simulink model "asadi_simulation"  (R2024b)
settings: Solver=VariableStepAuto  StartTime=0.0  StopTime=10  FixedStep=0.01  RelTol=1e-3
model workspace (MAT data in the model file):
  I_L = Simulink.Parameter
  I_L.Value = 0.0696
  I_L.Complexity = 'real'
  I_L.Dimensions = [1 1]
  I_L.DataType = 'auto'
  L = Simulink.Parameter
  L.Value = 0.375
  L.Complexity = 'real'
  L.Dimensions = [1 1]
  L.DataType = 'auto'
  M_EE = Simulink.Parameter
  M_EE.Value = 1.542
  M_EE.Complexity = 'real'
  M_EE.Dimensions = [1 1]
  M_EE.DataType = 'auto'
  M_L = Simulink.Parameter
  M_L.Value = 1.696
  M_L.Complexity = 'real'
  M_L.Dimensions = [1 1]
  M_L.DataType = 'auto'
  M_l = Simulink.Parameter
  M_l.Value = 0.334
  M_l.Complexity = 'real'
  M_l.Dimensions = [1 1]
  M_l.DataType = 'auto'
  l = Simulink.Parameter
  l.Value = 0.96
  l.Complexity = 'real'
  l.Dimensions = [1 1]
  l.DataType = 'auto'
undefined symbols (not defined in the file): i_L, l_L, l_l, m_EE, m_L, m_l
libraries: simulink x3
settings Model: Creator=marius  LastModifiedBy=marius
settings RTWCC: GPUComputeCapability=3.5

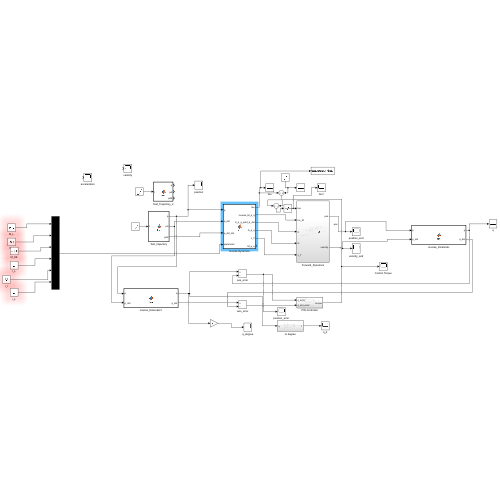
[thumbnail: Simulink's stored preview of the top-level diagram]
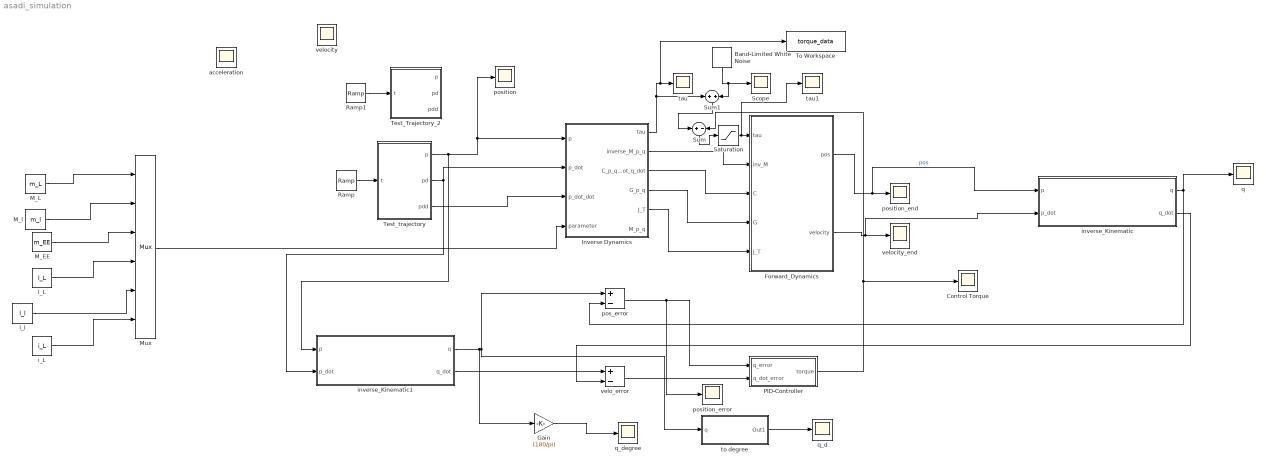
== system asadi_simulation ==
  Band-Limited White Noise : simulink/Sources/Band-Limited White Noise  Cov=[0.0005]  Ts=0.1  seed=[23341]
  Control Torque : Scope
  Forward_Dynamics : Subsystem
  Gain : Gain  Gain=(180/pi)
  Inverse Dynamics : MATLAB Function  TreatAsAtomicUnit=on
  M_EE : Constant  Value=m_EE
  M_L : Constant  Value=m_L
  M_l : Constant  Value=m_l
  Mux : Mux  Inputs=6
  PID-Controller : Subsystem
  Ramp : simulink/Sources/Ramp  slope=1  start=0  InitialOutput=0
  Ramp1 : simulink/Sources/Ramp  slope=1  start=0  InitialOutput=0
  Saturation : Saturate  UpperLimit=26  LowerLimit=-26
  Scope : Scope
  Sum : Sum  Inputs=+-
  Sum1 : Sum
  Test_Trajectory_2 : MATLAB Function  TreatAsAtomicUnit=on
  Test_trajectory : MATLAB Function  TreatAsAtomicUnit=on
  To Workspace : ToWorkspace  VariableName=torque_data  SaveFormat=Timeseries  SampleTime=-1
  acceleration : Scope
  i_L : Constant  Value=i_L
  inverse_Kinematic : MATLAB Function  TreatAsAtomicUnit=on
  inverse_Kinematic1 : MATLAB Function  TreatAsAtomicUnit=on
  l_L : Constant  Value=l_L
  l_l : Constant  Value=l_l
  pos_error : Sum  Inputs=+-
  position : Scope
  position_end : Scope
  position_error : Scope
  q : Scope
  q_d : Scope
  q_degree : Scope
  tau : Scope
  tau1 : Scope
  to degree : Subsystem
  velo_error : Sum  Inputs=+-
  velocity : Scope
  velocity_end : Scope
  wires:
  Inverse Dynamics/1(tau) -> Sum1/1, To Workspace/1, tau/1
  Inverse Dynamics/2(inverse_M_p_q) -> Forward_Dynamics/2(inv_M)
  Inverse Dynamics/3(C_p_q_pdot_q_dot) -> Forward_Dynamics/3(C)
  Inverse Dynamics/4(G_p_q) -> Forward_Dynamics/4(G)
  Inverse Dynamics/5(J_T) -> Forward_Dynamics/5(J_T)
  Forward_Dynamics/1(pos) -> inverse_Kinematic/1(p), position_end/1  "pos"
  Forward_Dynamics/2(velocity) -> inverse_Kinematic/2(p_dot), velocity_end/1
  pos_error/1 -> position_error/1, PID-Controller/1(q_error)
  inverse_Kinematic1/2(q_dot) -> velo_error/1
  inverse_Kinematic/2(q_dot) -> velo_error/2
  inverse_Kinematic/1(q) -> q/1, pos_error/2
  inverse_Kinematic1/1(q) -> Gain/1, pos_error/1, to degree/1(q)
  velo_error/1 -> PID-Controller/2(q_dot_error)
  Gain/1 -> q_degree/1
  Band-Limited White Noise/1 -> Scope/1, Sum1/2
  Sum1/1 -> Sum/1
  Ramp/1 -> Test_trajectory/1(t)
  Sum/1 -> Saturation/1
  to degree/1(Out1) -> q_d/1
  Saturation/1 -> tau1/1, Forward_Dynamics/1(tau)
  PID-Controller/1(torque) -> Sum/2, Control Torque/1
  Ramp1/1 -> Test_Trajectory_2/1(t)
  Test_trajectory/1(p) -> inverse_Kinematic1/1(p), position/1, Inverse Dynamics/1(p)
  Test_trajectory/2(pd) -> inverse_Kinematic1/2(p_dot), Inverse Dynamics/2(p_dot)
  Test_trajectory/3(pdd) -> Inverse Dynamics/3(p_dot_dot)
  M_L/1 -> Mux/1
  M_l/1 -> Mux/2
  M_EE/1 -> Mux/3
  Mux/1 -> Inverse Dynamics/4(parameter)
  l_L/1 -> Mux/4
  l_l/1 -> Mux/5
  i_L/1 -> Mux/6

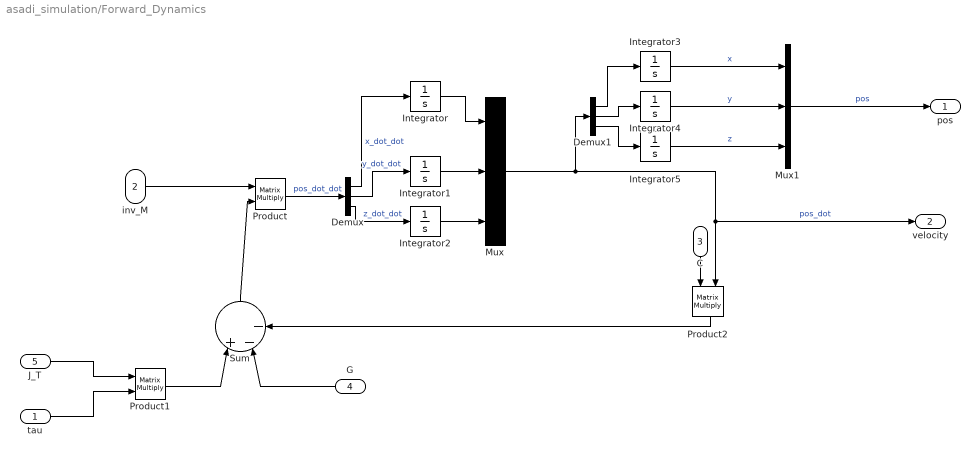
== system asadi_simulation/Forward_Dynamics ==
  tau : Inport
  inv_M : Inport  Port=2
  C : Inport  Port=3
  G : Inport  Port=4
  J_T : Inport  Port=5
  Demux : Demux  Outputs=3
  Demux1 : Demux  Outputs=3
  Integrator : Integrator  InitialCondition=0.4
  Integrator1 : Integrator  InitialCondition=0.8
  Integrator2 : Integrator  InitialCondition=0.8
  Integrator3 : Integrator
  Integrator4 : Integrator
  Integrator5 : Integrator  InitialCondition=-0.9
  Mux : Mux  Inputs=3
  Mux1 : Mux  Inputs=3
  Product : Product  Multiplication=Matrix(*)
  Product1 : Product  Multiplication=Matrix(*)
  Product2 : Product  Multiplication=Matrix(*)
  Sum : Sum  Inputs=|+--
  pos : Outport
  velocity : Outport  Port=2
  wires:
  inv_M/1 -> Product/1
  J_T/1 -> Product1/1
  tau/1 -> Product1/2
  Product1/1 -> Sum/1
  G/1 -> Sum/2
  Product2/1 -> Sum/3
  Sum/1 -> Product/2
  Product/1 -> Demux/1  "pos_dot_dot"
  Demux/3 -> Integrator2/1  "z_dot_dot"
  Demux/2 -> Integrator1/1  "y_dot_dot"
  Demux/1 -> Integrator/1  "x_dot_dot"
  Integrator2/1 -> Mux/3
  Integrator1/1 -> Mux/2
  Integrator/1 -> Mux/1
  Mux/1 -> velocity/1, Product2/2, Demux1/1  "pos_dot"
  Demux1/3 -> Integrator5/1
  Demux1/2 -> Integrator4/1
  Demux1/1 -> Integrator3/1
  Integrator5/1 -> Mux1/3  "z"
  Integrator4/1 -> Mux1/2  "y"
  Integrator3/1 -> Mux1/1  "x"
  Mux1/1 -> pos/1  "pos"
  C/1 -> Product2/1

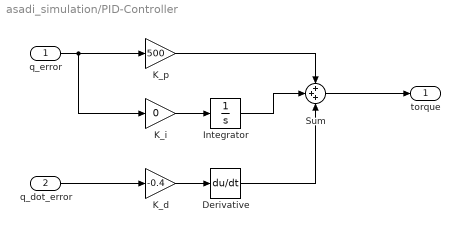
== system asadi_simulation/PID-Controller ==
  q_error : Inport
  q_dot_error : Inport  Port=2
  Derivative : Derivative
  Integrator : Integrator
  K_d : Gain  Gain=-0.4
  K_i : Gain  Gain=0
  K_p : Gain  Gain=500
  Sum : Sum  Inputs=+++
  torque : Outport
  wires:
  q_error/1 -> K_i/1, K_p/1
  K_p/1 -> Sum/1
  K_i/1 -> Integrator/1
  Integrator/1 -> Sum/2
  q_dot_error/1 -> K_d/1
  K_d/1 -> Derivative/1
  Derivative/1 -> Sum/3
  Sum/1 -> torque/1

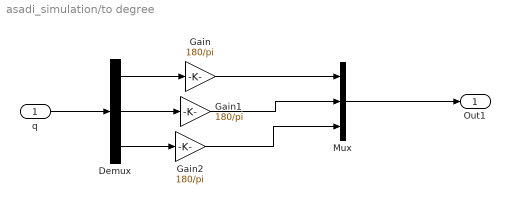
== system asadi_simulation/to degree ==
  q : Inport
  Demux : Demux  Outputs=3
  Gain : Gain  Gain=180/pi
  Gain1 : Gain  Gain=180/pi
  Gain2 : Gain  Gain=180/pi
  Mux : Mux  Inputs=3
  Out1 : Outport
  wires:
  q/1 -> Demux/1
  Demux/3 -> Gain2/1
  Gain2/1 -> Mux/3
  Demux/2 -> Gain1/1
  Demux/1 -> Gain/1
  Gain/1 -> Mux/1
  Gain1/1 -> Mux/2
  Mux/1 -> Out1/1

== matlab function asadi_simulation/Test_trajectory ==
  data: t input; p output; pd output; pdd output
function [p, pd, pdd] = fcn(t)
pos_x= sin(2*t) * 0.2;
pos_y= sin(4*t) * 0.2;
pos_z = -0.9 + sin (4*t) * 0.2;
vel_x = 0.4 * cos(2*t);
vel_y = 0.8 * cos(4*t);
vel_z = cos(4*t) * 0.8;
acc_x = -0.8 * sin(2*t);
acc_y = -3.2*sin(4*t);
acc_z = -3.2 * sin(4*t);

p= [pos_x; pos_y; pos_z];
pd = [vel_x; vel_y; vel_z];
pdd = [acc_x; acc_y; acc_z];

== matlab function asadi_simulation/Inverse Dynamics ==
  data: p input; tau output; p_dot input; p_dot_dot input; inverse_M_p_q output; C_p_q_pdot_q_dot output; G_p_q output; J_T output; M_p_q output; parameter input
function [tau, inverse_M_p_q, C_p_q_pdot_q_dot, G_p_q, J_T, M_p_q]    = fcn(p, p_dot, p_dot_dot, parameter)
r_p = 0.07; %m
% radius base platform
r_b = 0.25; %m
%length upper arm
L = parameter(4);%0.375; m
%length fore arm
l = parameter(5); %0.96; %m

% mass proximal link
m_L = parameter(1);%1.636 kg
% mass distal link
M_K = parameter(2); %0.334 kg

% mass end_effector
m_p = parameter(3); %1.542kg

%proximal link inertia
I_L = parameter(6);%0.0696 ;% kg m^2

g = [0; 0; -9.808]; % m/s^2
c = r_p - r_b;
x = p(1);
y = p(2);
z = p(3);
E1 = -(x + 2*c + sqrt(3)* y) * L;
E2 = -(x + 2*c - sqrt(3)* y) * L;
E3 = 2*(x-c)*L;

F1 = 2*z*L;
F2 = 2*z*L;
F3 = 2*z*L;

G1 = x^2 + y^2 + z^2 + c*x + c^2 + L^2 + sqrt(3)* c * y - l^2;
G2 = x^2 + y^2 + z^2 + c*x +c^2 + L^2 - sqrt(3)* c * y - l^2;
G3 = x^2 + y^2 + z^2 + c^2 -2*c*x + L^2 -l^2;

auxterm_1 = E1^2 + F1^2 - G1^2;
auxterm_2 = E2^2 + F2^2 - G2^2;
auxterm_3 = E3^2 + F3^2 - G3^2;

t_1_1 = (-F1 + sqrt(auxterm_1)) / (G1 - E1);
t_1_2 = (-F1 - sqrt(auxterm_1)) / (G1 - E1);

t_2_1 = (-F2 + sqrt(auxterm_2)) / (G2 - E2);
t_2_2 = (-F2 - sqrt(auxterm_2)) / (G2 - E2);

t_3_1 = (-F3 + sqrt(auxterm_3)) / (G3 - E3);
t_3_2 = (-F3 - sqrt(auxterm_3)) / (G3 - E3);

theta_1_1 = 2*atan(t_1_1);
theta_1_2 = 2*atan(t_1_2);
theta_1_1_deg = theta_1_1 * 180/pi;
theta_1_2_deg = theta_1_2 * 180/pi;

theta_2_1 = 2*atan(t_2_1);
theta_2_2 = 2*atan(t_2_2);
theta_2_1_deg = theta_2_1 * 180/pi;
theta_2_2_deg = theta_2_2 * 180/pi;

theta_3_1 = 2*atan(t_3_1);
theta_3_2 = 2*atan(t_3_2);
theta_3_1_deg = theta_3_1 * 180/pi;
theta_3_2_deg = theta_3_2 * 180/pi;


q1 = -theta_1_2;
q2 = -theta_2_2;
q3 = -theta_3_2; % minus because asadi uses another convention, q turns in negative direction

% Jacobians

R_b = [0; r_b; 0];
R_a = [0; r_p; 0];

phi_1 = -pi/6;
phi_2 = -5*pi/6;
phi_3 = pi/2;


rotation_R_1 = [cos(phi_1) -sin(phi_1) 0; sin(phi_1) cos(phi_1) 0; 0 0 1];
rotation_R_2 = [cos(phi_2) -sin(phi_2) 0; sin(phi_2) cos(phi_2) 0; 0 0 1];
rotation_R_3 = [cos(phi_3) -sin(phi_3) 0; sin(phi_3) cos(phi_3) 0; 0 0 1];

rotation_O_1 = [1 0 0; 0 cos(q1) -sin(q1); 0 sin(q1) cos(q1)];
rotation_O_2 = [1 0 0; 0 cos(q2) -sin(q2); 0 sin(q2) cos(q2)];
rotation_O_3 = [1 0 0; 0 cos(q3) -sin(q3); 0 sin(q3) cos(q3)];

%L vector along the positive y-Axis of the frame which moves with the upper
%arm
L_vec = [0; L; 0];
U_1 = p - rotation_R_1*((R_b - R_a) + rotation_O_1*L_vec);

U_2 = p - rotation_R_2*((R_b - R_a) + rotation_O_2*L_vec);
U_3 = p - rotation_R_3*((R_b - R_a) + rotation_O_3*L_vec);

S_1 = [0 0 0; 0 0 -1; 0 1 0];
T_1 = rotation_R_1 * S_1 * rotation_O_1* L_vec;
T_2 = rotation_R_2 * S_1 * rotation_O_2* L_vec;
T_3 = rotation_R_3 * S_1 * rotation_O_3* L_vec;


Jacobian = [U_1'*T_1, 0, 0; 0, U_2'*T_2, 0; 0, 0, U_3'*T_3] \ [U_1'; U_2'; U_3'];

%q_dot
q_dot = Jacobian * p_dot;


T_dot_1 = rotation_R_1*S_1 * S_1 * rotation_O_1* L_vec * q_dot(1);
T_dot_2 = rotation_R_2*S_1 * S_1 * rotation_O_2* L_vec * q_dot(2);
T_dot_3 = rotation_R_3*S_1 * S_1 * rotation_O_3* L_vec * q_dot(3);

U_dot_1 = p_dot - T_1 * q_dot(1);
U_dot_2 = p_dot - T_2 * q_dot(2);
U_dot_3 = p_dot - T_3 * q_dot(3);

inverse_Jacobian_aux = inv([U_1'*T_1, 0, 0; 0, U_2'*T_2, 0; 0, 0, U_3'*T_3]);
%another auxiliary vector
vec_1 = U_dot_1' - (U_dot_1' * T_1 + U_1'*T_dot_1)*Jacobian(1,:);
vec_2 = U_dot_2' - (U_dot_2' * T_2 + U_2'*T_dot_2)*Jacobian(2,:);
vec_3 = U_dot_3' - (U_dot_3' * T_3 + U_3'*T_dot_3)*Jacobian(3,:);

Jacobian_dot = cross(inverse_Jacobian_aux, [vec_1; vec_2; vec_3]);

omega_L_1 = [Jacobian(1,:); 0 0 0; 0 0 0] * p_dot;
omega_L_2 = [Jacobian(2,:); 0 0 0; 0 0 0] * p_dot;
omega_L_3 = [Jacobian(3,:); 0 0 0; 0 0 0] * p_dot;

r_L = 0.373; %proximal link length ratio COM
v_L_1 = cross(omega_L_1, r_L*[0;1;0]);
v_L_2 = cross(omega_L_2, r_L*[0;1;0]);
v_L_3 = cross(omega_L_3, r_L*[0;1;0]);

omega_L_dot_1 = [Jacobian(1,:); 0 0 0; 0 0 0]* p_dot_dot + [Jacobian_dot(1,:); 0 0 0; 0 0 0] * p_dot;
omega_L_dot_2 = [Jacobian(2,:); 0 0 0; 0 0 0]* p_dot_dot + [Jacobian_dot(2,:); 0 0 0; 0 0 0] * p_dot;
omega_L_dot_3 = [Jacobian(3,:); 0 0 0; 0 0 0]* p_dot_dot + [Jacobian_dot(3,:); 0 0 0; 0 0 0] * p_dot;

v_L_dot_1 = r_L * L * [0 0 0; 0 0 0; Jacobian(1,:)]* p_dot_dot + r_L * L *...
    [0 0 0; -p_dot' * Jacobian(1, :)' * Jacobian(1,:); Jacobian_dot(1,:)] * p_dot;
v_L_dot_2 = r_L * L * [0 0 0; 0 0 0; Jacobian(2,:)]* p_dot_dot + r_L * L *...
    [0 0 0; -p_dot' * Jacobian(2, :)' * Jacobian(2,:); Jacobian_dot(2,:)] * p_dot;
v_L_dot_3 = r_L * L * [0 0 0; 0 0 0; Jacobian(3,:)]* p_dot_dot + r_L * L *...
    [0 0 0; -p_dot' * Jacobian(3, :)' * Jacobian(3,:); Jacobian_dot(3,:)] * p_dot;
r_K = 0.5; % distal link length ratio COM

v_K_1 = ((1-r_K)*L*[0 0 0; 0 0 0; Jacobian(1,:)] + r_K * rotation_O_1' * rotation_R_1') * p_dot;
v_K_2 = ((1-r_K)*L*[0 0 0; 0 0 0; Jacobian(2,:)] + r_K * rotation_O_2' * rotation_R_2') * p_dot;
v_K_3 = ((1-r_K)*L*[0 0 0; 0 0 0; Jacobian(3,:)] + r_K * rotation_O_3' * rotation_R_3') * p_dot;

v_K_dot_1 = ((1-r_K)*L*[0 0 0; 0 0 0; Jacobian(1,:)] + r_K * rotation_O_1' * rotation_R_1') * p_dot_dot...
    + (1-r_K)* L * [0 0 0; - p_dot' * Jacobian(1,:)' * Jacobian(1,:); Jacobian_dot(1,:)]* p_dot;

v_K_dot_2 = ((1-r_K)*L*[0 0 0; 0 0 0; Jacobian(2,:)] + r_K * rotation_O_2' * rotation_R_2') * p_dot_dot...
    + (1-r_K)* L * [0 0 0; - p_dot' * Jacobian(2,:)' * Jacobian(2,:); Jacobian_dot(2,:)]* p_dot;

v_K_dot_3 = ((1-r_K)*L*[0 0 0; 0 0 0; Jacobian(3,:)] + r_K * rotation_O_3' * rotation_R_3') * p_dot_dot...
    + (1-r_K)* L * [0 0 0; - p_dot' * Jacobian(3,:)' * Jacobian(3,:); Jacobian_dot(3,:)]* p_dot;


% auxiliary Jacobians
J_L_1 = r_L * L * [0 0 0; 0 0 0; Jacobian(1,:)];
J_L_2 = r_L * L * [0 0 0; 0 0 0; Jacobian(2,:)];
J_L_3 = r_L * L * [0 0 0; 0 0 0; Jacobian(3,:)];

J_K_1 = (1-r_K)* L* [0 0 0; 0 0 0; Jacobian(1,:)] + r_K *rotation_O_1' * rotation_R_1';
J_K_2 = (1-r_K)* L* [0 0 0; 0 0 0; Jacobian(2,:)] + r_K *rotation_O_2' * rotation_R_2';
J_K_3 = (1-r_K)* L* [0 0 0; 0 0 0; Jacobian(3,:)] + r_K *rotation_O_3' * rotation_R_3';

J_C_1 = L * [0 0 0; 0 0 0; Jacobian(1,:)];
J_C_2 = L * [0 0 0; 0 0 0; Jacobian(2,:)];
J_C_3 = L * [0 0 0; 0 0 0; Jacobian(3,:)];


% distal link dominant inertia
I_K = 0.00057; %kg m^2
% Inertia motor
I_Mo = 0.0465;


% mass distributions
A = [1 1 1; r_K (r_K-1) 0; r_K^2*l^2 (r_K-1)^2 *l^2 0];
b_vec = [M_K; 0; I_K];
x = A\b_vec;
% mass distributed to elbow
m_c = x(1);
% mass distributed to endeffector
m_A = x(2);
% mass distributed to COM distal link
m_K = x(3);

identity = eye(3);


% Massmatrix 

sum_one = m_K* r_K * J_K_1' * rotation_O_1' * rotation_R_1'...
    + m_K * r_K * J_K_2'*rotation_O_2'* rotation_R_2' + m_K* r_K * J_K_3' * rotation_O_3' * rotation_R_3';
sum_two_one = (m_c*L*J_C_1' + m_L * r_L * L * J_L_1' + m_K*(1-r_K)*L*J_K_1') * [0 0 0; 0 0 0; Jacobian(1,:)];
sum_two_two = (m_c*L*J_C_2' + m_L * r_L * L * J_L_2' + m_K*(1-r_K)*L*J_K_2') * [0 0 0; 0 0 0; Jacobian(2,:)];
sum_two_three = (m_c*L*J_C_3' + m_L * r_L * L * J_L_3' + m_K*(1-r_K)*L*J_K_3') * [0 0 0; 0 0 0; Jacobian(3,:)];
sum_two = sum_two_one + sum_two_two + sum_two_three;
M_p_q = (I_Mo +  I_L) * (Jacobian' * Jacobian) + (m_p + 3*m_c)* identity + sum_one + sum_two;


% matrix of coriolis and centrifugal forces
sum_c = (m_c*L*J_C_1' + m_L*r_L*L * J_L_1' + m_K*(1-r_K)*L*J_K_1') * [0 0 0; -p_dot' *Jacobian(1,:)' * Jacobian(1,:); Jacobian_dot(1,:)]...
    +(m_c*L*J_C_2' + m_L*r_L*L * J_L_2' + m_K*(1-r_K)*L*J_K_2') * [0 0 0; -p_dot' *Jacobian(2,:)' * Jacobian(2,:); Jacobian_dot(2,:)]...
    +(m_c*L*J_C_3' + m_L*r_L*L * J_L_3' + m_K*(1-r_K)*L*J_K_3') * [0 0 0; -p_dot' *Jacobian(3,:)' * Jacobian(3,:); Jacobian_dot(3,:)];
C_p_q_pdot_q_dot = (I_Mo + I_L)* Jacobian' * Jacobian_dot + sum_c;


sum_g = ((m_c* J_C_1' + m_L*J_L_1' + m_K* J_K_1') * rotation_O_1' * rotation_R_1')*g ...
    + ((m_c* J_C_2' + m_L*J_L_2' + m_K* J_K_2') * rotation_O_2' * rotation_R_2')*g ...
    + ((m_c* J_C_3' + m_L*J_L_3' + m_K* J_K_3') * rotation_O_3' * rotation_R_3')*g;

G_p_q = -(m_p + 3* m_A) * g - sum_g;
inverse_M_p_q = inv(M_p_q);
J_T = Jacobian';
F_p = 0;
motion_equation =  M_p_q * p_dot_dot + C_p_q_pdot_q_dot * p_dot + G_p_q - F_p;
tau =  J_T\ motion_equation;

== matlab function asadi_simulation/inverse_Kinematic ==
  data: p input; q output; p_dot input; q_dot output
function [q, q_dot] = fcn(p, p_dot)

% radius moving platform
r_p = 0.07; %m
% radius base platform
r_b = 0.25; %m
%length upper arm
L = 0.375; %m
%length fore arm
l = 0.96; %m

c = r_p - r_b;
x = p(1);
y = p(2);
z = p(3);

E1 = -(x + 2*c + sqrt(3)* y) * L;
E2 = -(x + 2*c - sqrt(3)* y) * L;
E3 = 2*(x-c)*L;

F1 = 2*z*L;
F2 = 2*z*L;
F3 = 2*z*L;

abs_pos = x^2 + y^2 + z^2;
G1 = abs_pos + c*x + c^2 + L^2 + sqrt(3)* c * y - l^2;
G2 = abs_pos + c*x +c^2 + L^2 - sqrt(3)* c * y - l^2;
G3 = abs_pos + c^2 -2*c*x + L^2 -l^2;


%auxiliary term
aux_T_1 = sqrt(E1^2 + F1^2 - G1^2);
aux_T_2 = sqrt(E2^2 + F2^2 - G2^2);
aux_T_3 = sqrt(E3^2 + F3^2 - G3^2);
%quadratic formula.
t_1_1 = (-F1 + aux_T_1) / (G1 - E1);
t_1_2 = (-F1 - aux_T_1) / (G1 - E1);

t_2_1 = (-F2 + aux_T_2) / (G2 - E2);
t_2_2 = (-F2 - aux_T_2) / (G2 - E2);

t_3_1 = (-F3 + aux_T_3) / (G3 - E3);
t_3_2 = (-F3 - aux_T_3) / (G3 - E3);

theta_1_1 = 2*atan(t_1_1);
theta_1_2 = 2*atan(t_1_2);


theta_2_1 = 2*atan(t_2_1);
theta_2_2 = 2*atan(t_2_2);

theta_3_1 = 2*atan(t_3_1);
theta_3_2 = 2*atan(t_3_2);


q1 = -theta_1_2;
q2 = -theta_2_2;
q3 = -theta_3_2;
% using the negative because of different convention
q=-[q1; q2; q3];
% Jacobians

R_b = [0; r_b; 0];
R_a = [0; r_p; 0];
phi_1 = -pi/6;
phi_2 = -5*pi/6;
phi_3 = pi/2;
rotation_R_1 = [cos(phi_1) -sin(phi_1) 0; sin(phi_1) cos(phi_1) 0; 0 0 1];
rotation_R_2 = [cos(phi_2) -sin(phi_2) 0; sin(phi_2) cos(phi_2) 0; 0 0 1];
rotation_R_3 = [cos(phi_3) -sin(phi_3) 0; sin(phi_3) cos(phi_3) 0; 0 0 1];

rotation_O_1 = [1 0 0; 0 cos(q1) -sin(q1); 0 sin(q1) cos(q1)];
rotation_O_2 = [1 0 0; 0 cos(q2) -sin(q2); 0 sin(q2) cos(q2)];
rotation_O_3 = [1 0 0; 0 cos(q3) -sin(q3); 0 sin(q3) cos(q3)];

%L vector along the positive y-Axis of the frame which moves with the upper
%arm
L_vec = [0; L; 0];
U_1 = p - rotation_R_1*((R_b - R_a) + rotation_O_1*L_vec);

U_2 = p - rotation_R_2*((R_b - R_a) + rotation_O_2*L_vec);
U_3 = p - rotation_R_3*((R_b - R_a) + rotation_O_3*L_vec);

S_1 = [0 0 0; 0 0 -1; 0 1 0];
T_1 = rotation_R_1 * S_1 * rotation_O_1* L_vec;
T_2 = rotation_R_2 * S_1 * rotation_O_2* L_vec;
T_3 = rotation_R_3 * S_1 * rotation_O_3* L_vec;


Jacobian = [U_1'*T_1, 0, 0; 0, U_2'*T_2, 0; 0, 0, U_3'*T_3] \ [U_1'; U_2'; U_3'];

%q_dot
q_dot = Jacobian * p_dot;

== matlab function asadi_simulation/inverse_Kinematic1 ==
  data: p input; q output; p_dot input; q_dot output
function [q, q_dot] = fcn(p, p_dot)

% radius moving platform
r_p = 0.07; %m
% radius base platform
r_b = 0.25; %m
%length upper arm
L = 0.375; %m
%length fore arm
l = 0.96; %m

c = r_p - r_b;
x = p(1);
y = p(2);
z = p(3);

E1 = -(x + 2*c + sqrt(3)* y) * L;
E2 = -(x + 2*c - sqrt(3)* y) * L;
E3 = 2*(x-c)*L;

F1 = 2*z*L;
F2 = 2*z*L;
F3 = 2*z*L;

abs_pos = x^2 + y^2 + z^2;
G1 = abs_pos + c*x + c^2 + L^2 + sqrt(3)* c * y - l^2;
G2 = abs_pos + c*x +c^2 + L^2 - sqrt(3)* c * y - l^2;
G3 = abs_pos + c^2 -2*c*x + L^2 -l^2;


%auxiliary term
aux_T_1 = sqrt(E1^2 + F1^2 - G1^2);
aux_T_2 = sqrt(E2^2 + F2^2 - G2^2);
aux_T_3 = sqrt(E3^2 + F3^2 - G3^2);
%quadratic formula.
t_1_1 = (-F1 + aux_T_1) / (G1 - E1);
t_1_2 = (-F1 - aux_T_1) / (G1 - E1);

t_2_1 = (-F2 + aux_T_2) / (G2 - E2);
t_2_2 = (-F2 - aux_T_2) / (G2 - E2);

t_3_1 = (-F3 + aux_T_3) / (G3 - E3);
t_3_2 = (-F3 - aux_T_3) / (G3 - E3);

theta_1_1 = 2*atan(t_1_1);
theta_1_2 = 2*atan(t_1_2);


theta_2_1 = 2*atan(t_2_1);
theta_2_2 = 2*atan(t_2_2);

theta_3_1 = 2*atan(t_3_1);
theta_3_2 = 2*atan(t_3_2);


q1 = -theta_1_2;
q2 = -theta_2_2;
q3 = -theta_3_2;
% using the negative because of different convention
q=-[q1; q2; q3];
% Jacobians

R_b = [0; r_b; 0];
R_a = [0; r_p; 0];
phi_1 = -pi/6;
phi_2 = -5*pi/6;
phi_3 = pi/2;
rotation_R_1 = [cos(phi_1) -sin(phi_1) 0; sin(phi_1) cos(phi_1) 0; 0 0 1];
rotation_R_2 = [cos(phi_2) -sin(phi_2) 0; sin(phi_2) cos(phi_2) 0; 0 0 1];
rotation_R_3 = [cos(phi_3) -sin(phi_3) 0; sin(phi_3) cos(phi_3) 0; 0 0 1];

rotation_O_1 = [1 0 0; 0 cos(q1) -sin(q1); 0 sin(q1) cos(q1)];
rotation_O_2 = [1 0 0; 0 cos(q2) -sin(q2); 0 sin(q2) cos(q2)];
rotation_O_3 = [1 0 0; 0 cos(q3) -sin(q3); 0 sin(q3) cos(q3)];

%L vector along the positive y-Axis of the frame which moves with the upper
%arm
L_vec = [0; L; 0];
U_1 = p - rotation_R_1*((R_b - R_a) + rotation_O_1*L_vec);

U_2 = p - rotation_R_2*((R_b - R_a) + rotation_O_2*L_vec);
U_3 = p - rotation_R_3*((R_b - R_a) + rotation_O_3*L_vec);

S_1 = [0 0 0; 0 0 -1; 0 1 0];
T_1 = rotation_R_1 * S_1 * rotation_O_1* L_vec;
T_2 = rotation_R_2 * S_1 * rotation_O_2* L_vec;
T_3 = rotation_R_3 * S_1 * rotation_O_3* L_vec;


Jacobian = [U_1'*T_1, 0, 0; 0, U_2'*T_2, 0; 0, 0, U_3'*T_3] \ [U_1'; U_2'; U_3'];

%q_dot
q_dot = Jacobian * p_dot;

== matlab function asadi_simulation/Test_Trajectory_2 ==
  data: t input; p output; pd output; pdd output
function [p, pd, pdd] = fcn(t)
pos_x= 0.25* cos(t);
pos_y= 0.25* sin(t);
pos_z = -0.9;
vel_x = -0.25 * sin(t);
vel_y = 0.25 * cos(t);
vel_z = 0;
acc_x = -0.25 * cos(t);
acc_y = -0.25*sin(t);
acc_z = 0;

p= [pos_x; pos_y; pos_z];
pd = [vel_x; vel_y; vel_z];
pdd = [acc_x; acc_y; acc_z];
